simulink model "EPD_5_gen_without_limits_dell_p_values"  (R2021b)
settings: Solver=VariableStepAuto  StartTime=0.0  StopTime=10.0  RelTol=1e-3
settings Model: Creator=vijay  LastModifiedBy=vijay

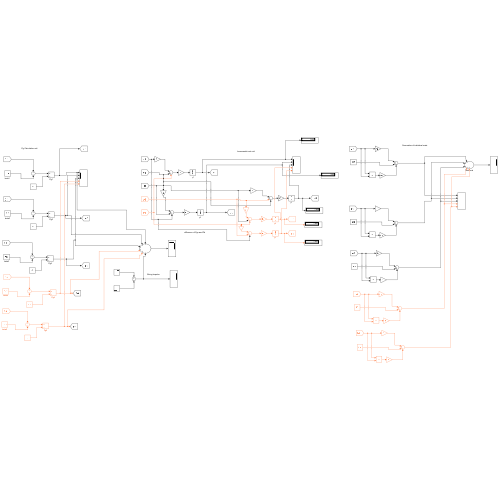
[thumbnail: Simulink's stored preview of the top-level diagram]
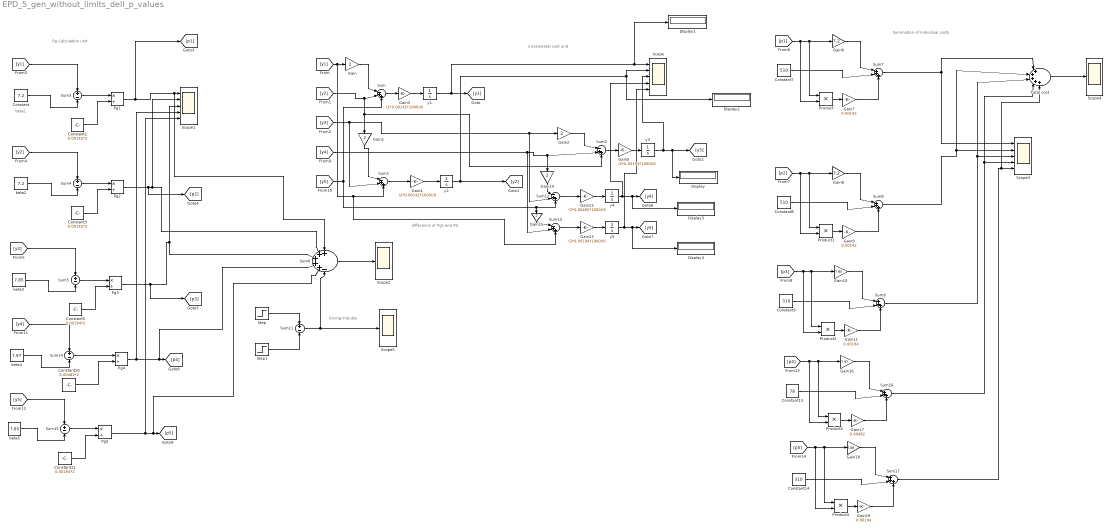
== system EPD_5_gen_without_limits_dell_p_values ==
  note: beta1
  note: Giving Impulse
  note: Pg Calculation unit
  note: Incremental cost unit
  note: Summation of individual costs
  note: difference of Pgs and Pd
  Constant : Constant  Value=7.2
  Constant1 : Constant  Value=0.00142*2
  Constant10 : Constant  Value=0.00482*2
  Constant11 : Constant  Value=0.00194*2
  Constant13 : Constant  Value=78
  Constant14 : Constant  Value=310
  Constant3 : Constant  Value=0.00142*2
  Constant5 : Constant  Value=0.00194*2
  Constant7 : Constant  Value=510
  Constant8 : Constant  Value=510
  Constant9 : Constant  Value=310
  Display{,1..4} (5 alike) : Display
  Gain{,1..2,14..15} (5 alike) : Gain  Gain=2
  Gain10 : Gain  Gain=7.85
  Gain11 : Gain  Gain=0.00194
  Gain12 : Gain  Gain=(2*0.00482*1000)/6
  Gain13 : Gain  Gain=(2*0.00194*1000)/6
  Gain16 : Gain  Gain=7.97
  Gain17 : Gain  Gain=0.00482
  Gain18 : Gain  Gain=7.85
  Gain19 : Gain  Gain=0.00194
  Gain3 : Gain  Gain=(2*0.00142*1000)/6
  Gain4 : Gain  Gain=(2*0.00142*1000)/6
  Gain5 : Gain  Gain=(2*0.00194*1000)/6
  Gain6 : Gain  Gain=7.2
  Gain7 : Gain  Gain=0.00142
  Gain8 : Gain  Gain=7.2
  Gain9 : Gain  Gain=0.00142
  Pg{1..5} (5 alike) : Product  Inputs=*/
  Product{,1..4} (5 alike) : Product
  Scope : Scope  NumInputPorts=5
  Scope1 : Scope  NumInputPorts=5
  Scope2 : Scope
  Scope3 : Scope  NumInputPorts=5
  Scope4 : Scope
  Scope5 : Scope
  Step : Step  Time=0.025  After=650  SampleTime=0
  Step1 : Step  Time=0.05  After=650  SampleTime=0
  Sum{,1..2,12..13} (5 alike) : Sum  Inputs=|-++
  Sum{3..5,11,14..15} (6 alike) : Sum  Inputs=+-
  Sum{7..9,16..17} (5 alike) : Sum  Inputs=|+++
  Sum6 : Sum  Inputs=+++++-
  Total cost : Sum  Inputs=|+++++
  beta2 : Constant  Value=7.2
  beta3 : Constant  Value=7.85
  beta4 : Constant  Value=7.97
  beta5 : Constant  Value=7.85
  y1 : Integrator  InitialCondition=7.626
  y2 : Integrator  InitialCondition=7.626
  y3 : Integrator  InitialCondition=8.238
  y4 : Integrator  InitialCondition=8.452
  y5 : Integrator  InitialCondition=8.238
  wires:
  Sum11/1 -> Scope5/1, Sum6/6
  Gain4/1 -> y2/1
  Sum2/1 -> Gain5/1
  Gain7/1 -> Sum7/3
  Step1/1 -> Sum11/2
  Step/1 -> Sum11/1
  Constant3/1 -> Pg2/2
  [y1] -> Sum3/1
  Gain11/1 -> Sum9/3
  Sum7/1 -> Scope3/1, Total cost/1
  Gain10/1 -> Sum9/1
  Total cost/1 -> Scope4/1
  [y2] -> Sum4/1
  Constant7/1 -> Sum7/2
  Constant9/1 -> Sum9/2
  Product2/1 -> Gain11/1
  [y3] -> Sum1/2, Sum12/2, Gain2/1
  Sum9/1 -> Total cost/3, Scope3/3
  [p2] -> Product1/2, Product1/1, Gain8/1
  Gain5/1 -> y3/1
  [p1] -> Product/2, Product/1, Gain6/1
  Product1/1 -> Gain9/1
  Gain1/1 -> Sum1/1
  [y1] -> Sum1/3, Sum13/3, Gain/1
  Pg1/1 -> [p1], Sum6/1, Scope1/1
  Gain/1 -> Sum/1
  Gain9/1 -> Sum8/3
  Sum5/1 -> Pg3/1
  Pg3/1 -> [p3], Scope1/3, Sum6/3
  Gain3/1 -> y1/1
  Product/1 -> Gain7/1
  Sum6/1 -> Scope2/1
  Gain6/1 -> Sum7/1
  Pg2/1 -> [p2], Scope1/2, Sum6/2
  Sum3/1 -> Pg1/1
  Constant5/1 -> Pg3/2
  beta3/1 -> Sum5/2
  [y2] -> Sum2/3, Gain1/1, Sum/2
  y3/1 -> Scope/3, Display/1, [y3]
  Constant/1 -> Sum3/2
  Sum/1 -> Gain3/1
  Sum4/1 -> Pg2/1
  Gain8/1 -> Sum8/1
  Constant1/1 -> Pg1/2
  Constant8/1 -> Sum8/2
  Sum8/1 -> Total cost/2, Scope3/2
  [y3] -> Sum5/1
  Gain2/1 -> Sum2/1
  y1/1 -> Display1/1, Scope/1, [y1]
  beta2/1 -> Sum4/2
  Sum1/1 -> Gain4/1
  [p3] -> Product2/2, Product2/1, Gain10/1
  y2/1 -> [y2], Display2/1, Scope/2
  [y5] -> Gain15/1, Sum12/3, Sum/3
  [y4] -> Sum13/2, Gain14/1, Sum2/2
  y4/1 -> Display3/1, [y4], Scope/4
  Gain12/1 -> y4/1
  Sum12/1 -> Gain12/1
  Gain14/1 -> Sum12/1
  Sum13/1 -> Gain13/1
  Gain13/1 -> y5/1
  y5/1 -> Scope/5, Display4/1, [y5]
  Gain15/1 -> Sum13/1
  [y4] -> Sum14/1
  beta4/1 -> Sum14/2
  Constant10/1 -> Pg4/2
  Sum14/1 -> Pg4/1
  Sum15/1 -> Pg5/1
  Constant11/1 -> Pg5/2
  beta5/1 -> Sum15/2
  [y5] -> Sum15/1
  Pg4/1 -> Scope1/4, Sum6/4, [p4]
  Pg5/1 -> Scope1/5, Sum6/5, [p5]
  [p4] -> Gain16/1, Product3/1, Product3/2
  Product3/1 -> Gain17/1
  Constant13/1 -> Sum16/2
  Gain16/1 -> Sum16/1
  Gain17/1 -> Sum16/3
  Gain19/1 -> Sum17/3
  Gain18/1 -> Sum17/1
  Constant14/1 -> Sum17/2
  Product4/1 -> Gain19/1
  [p5] -> Product4/2, Product4/1, Gain18/1
  Sum16/1 -> Scope3/4, Total cost/4
  Sum17/1 -> Total cost/5, Scope3/5
